simulink model "mrefrobotarm_modified_previous_y_previous_u_previous_ref_pert"  (R2018b)
settings: Solver=FixedStepAuto  StartTime=0.0  StopTime=10  RelTol=1e-3  AbsTol=1e-6
undefined symbols (not defined in the file or in its folder): cc, options
libraries: neural x714, simulink x1
(part 11 of 26)

== system mrefrobotarm_modified_previous_y_previous_u_previous_ref_pert/m=0.01 sd=0.001/Layer 3/Delays 1 ==
  "p{3}" : Inport  PortDimensions=30
      mask Display: e = 0.06;c1 = [120 230 180]/255;c2 = ([120 230 180]+0)/(256+128);c3 = ([120 230 180]+128)/(256+128);patch([0 1 1 0],[0 0 1 1],c1);patch([0 1 1 1-e 1-e 0+e],[0 0 1 1-e 0+e 0+e],c2);patch([0 0 1 1-e 0+e 0+e],[0 1 1 1-e 1-e 0+e],c3);plot([0 1 1 0 0],[0 0 1 1 0]);
  mux : Mux  Inputs=1
      mask Display: e = 0.06;c1 = [120 150 230]/255;c2 = ([120 150 230]+0)/383;c3 = ([120 150 230]+128)/383;patch([0 1 1 0],[0 0 1 1],c1);patch([0 1 1 1-e 1-e 0+e],[0 0 1 1-e 0+e 0+e],c2);patch([0 0 1 1-e 0+e 0+e],[0 1 1 1-e 1-e 0+e],c3);plot([0 1 1 0 0],[0 0 1 1 0]);disp('Mux')
  "pd{3,2}" : Outport
      mask Display: e = 0.06;c1 = [120 230 180]/255;c2 = ([120 230 180]+0)/(256+128);c3 = ([120 230 180]+128)/(256+128);patch([0 1 1 0],[0 0 1 1],c1);patch([0 1 1 1-e 1-e 0+e],[0 0 1 1-e 0+e 0+e],c2);patch([0 0 1 1-e 0+e 0+e],[0 1 1 1-e 1-e 0+e],c3);plot([0 1 1 0 0],[0 0 1 1 0]);
  wires:
  "p{3}"/1 -> mux/1
  mux/1 -> "pd{3,2}"/1

== system mrefrobotarm_modified_previous_y_previous_u_previous_ref_pert/m=0.01 sd=0.001/Layer 3/LW{3,2} ==
  "ad{3,2}" : Inport  PortDimensions=30
      mask Display: e = 0.06;c1 = [120 230 180]/255;c2 = ([120 230 180]+0)/(256+128);c3 = ([120 230 180]+128)/(256+128);patch([0 1 1 0],[0 0 1 1],c1);patch([0 1 1 1-e 1-e 0+e],[0 0 1 1-e 0+e 0+e],c2);patch([0 0 1 1-e 0+e 0+e],[0 1 1 1-e 1-e 0+e],c3);plot([0 1 1 0 0],[0 0 1 1 0]);
  "IW{3,2}(1,:)'" : Constant  Value=[-0.04154814424599621858202880275712232105433940887451171875;-0.0728322351099826847953266906188218854367733001708984375;0.08806929595322621207031943413312546908855438232421875;-0.06181152843373451111208538577557192184031009674072265625;0.05066544886284578275148504644675995223224163055419921875;0.111521575638174275102443289142684079706668853759765625;-0.032112539789640813514548511875545955263078212738037109375;-0.09799349563512209371207717367724399082362651824951171875;0.226222966133449665537824557759449817240238189697265625;-0.0164700269768449925056330584993702359497547149658203125;0.04924878083891880142797248254282749257981777191162109375;-0.31921274972881630294097021760535426437854766845703125;-0.00070955583482500985369190171780928722000680863857269287109375;-0.425499471575058574313032977443072013556957244873046875;-0.30280703571454103961713144599343650043010711669921875;0.020067038188739651227709970271462225355207920074462890625;0.1462301290259256092429751561212469823658466339111328125;0.204274950610219274693690749700181186199188232421875;-0.012345728106829323422743982519023120403289794921875;0.0182316153346177879657208364960752078332006931304931640625;0.1573963175042620010746219350039609707891941070556640625;-0.22786801020675173656826473234104923903942108154296875;-0.06417233312441379677881769794112187810242176055908203125;-0.044370962457045200200145274038732168264687061309814453125;-0.00712369940730364463454815648901785607449710369110107421875;-0.0964821250810107555739847384757013060152530670166015625;0.003950927495288344103163691301006110734306275844573974609375;0.11259508544268000129751072790895705111324787139892578125;-0.1494345742049391356776055772570543922483921051025390625;0.1954892809834287703552035964094102382659912109375]
      mask Display: e = 0.06;c1 = [120 150 230]/255;c2 = ([120 150 230]+0)/383;c3 = ([120 150 230]+128)/383;patch([0 1 1 0],[0 0 1 1],c1);patch([0 1 1 1-e 1-e 0+e],[0 0 1 1-e 0+e 0+e],c2);patch([0 0 1 1-e 0+e 0+e],[0 1 1 1-e 1-e 0+e],c3);plot([0 1 1 0 0],[0 0 1 1 0]);disp('weights');
  Mux : Mux  Inputs=1
      mask Display: e = 0.06;c1 = [120 150 230]/255;c2 = ([120 150 230]+0)/383;c3 = ([120 150 230]+128)/383;patch([0 1 1 0],[0 0 1 1],c1);patch([0 1 1 1-e 1-e 0+e],[0 0 1 1-e 0+e 0+e],c2);patch([0 0 1 1-e 0+e 0+e],[0 1 1 1-e 1-e 0+e],c3);plot([0 1 1 0 0],[0 0 1 1 0]);disp('Mux');
  dotprod1 : neural/Weight Functions/dotprod
  "lz{3,2}" : Outport
      mask Display: e = 0.06;c1 = [120 230 180]/255;c2 = ([120 230 180]+0)/(256+128);c3 = ([120 230 180]+128)/(256+128);patch([0 1 1 0],[0 0 1 1],c1);patch([0 1 1 1-e 1-e 0+e],[0 0 1 1-e 0+e 0+e],c2);patch([0 0 1 1-e 0+e 0+e],[0 1 1 1-e 1-e 0+e],c3);plot([0 1 1 0 0],[0 0 1 1 0]);
  wires:
  "IW{3,2}(1,:)'"/1 -> dotprod1/1
  "ad{3,2}"/1 -> dotprod1/2
  dotprod1/1 -> Mux/1
  Mux/1 -> "lz{3,2}"/1

== system mrefrobotarm_modified_previous_y_previous_u_previous_ref_pert/m=0.1 sd=0.1/Layer 1/Delays 1 ==
  "p{1}" : Inport  PortDimensions=10
      mask Display: e = 0.06;c1 = [120 230 180]/255;c2 = ([120 230 180]+0)/(256+128);c3 = ([120 230 180]+128)/(256+128);patch([0 1 1 0],[0 0 1 1],c1);patch([0 1 1 1-e 1-e 0+e],[0 0 1 1-e 0+e 0+e],c2);patch([0 0 1 1-e 0+e 0+e],[0 1 1 1-e 1-e 0+e],c3);plot([0 1 1 0 0],[0 0 1 1 0]);
  mux : Mux  Inputs=1
      mask Display: e = 0.06;c1 = [120 150 230]/255;c2 = ([120 150 230]+0)/383;c3 = ([120 150 230]+128)/383;patch([0 1 1 0],[0 0 1 1],c1);patch([0 1 1 1-e 1-e 0+e],[0 0 1 1-e 0+e 0+e],c2);patch([0 0 1 1-e 0+e 0+e],[0 1 1 1-e 1-e 0+e],c3);plot([0 1 1 0 0],[0 0 1 1 0]);disp('Mux')
  "pd{1,1}" : Outport
      mask Display: e = 0.06;c1 = [120 230 180]/255;c2 = ([120 230 180]+0)/(256+128);c3 = ([120 230 180]+128)/(256+128);patch([0 1 1 0],[0 0 1 1],c1);patch([0 1 1 1-e 1-e 0+e],[0 0 1 1-e 0+e 0+e],c2);patch([0 0 1 1-e 0+e 0+e],[0 1 1 1-e 1-e 0+e],c3);plot([0 1 1 0 0],[0 0 1 1 0]);
  wires:
  "p{1}"/1 -> mux/1
  mux/1 -> "pd{1,1}"/1

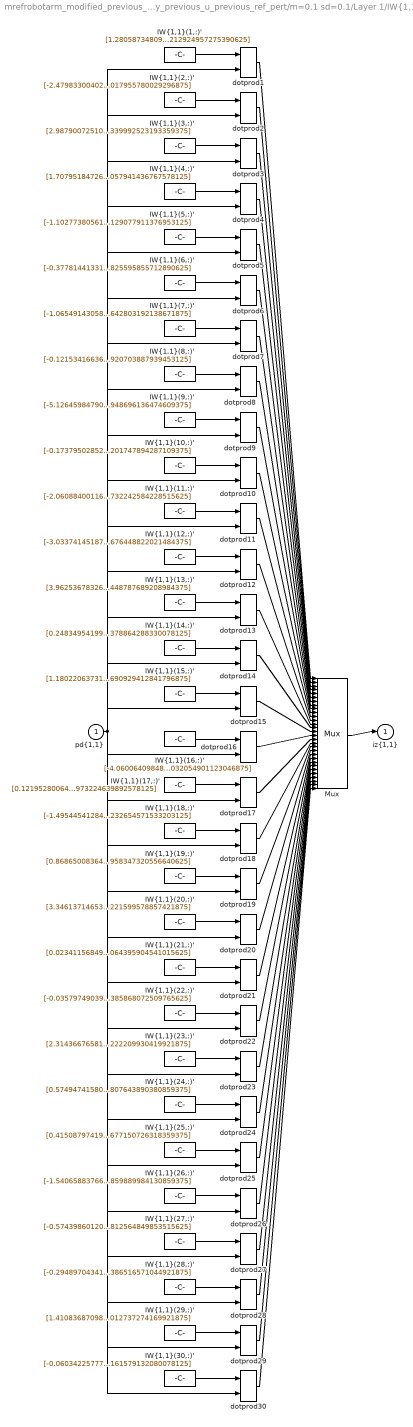
== system mrefrobotarm_modified_previous_y_previous_u_previous_ref_pert/m=0.1 sd=0.1/Layer 1/IW{1,1} ==
  "pd{1,1}" : Inport  PortDimensions=10
      mask Display: e = 0.06;c1 = [120 230 180]/255;c2 = ([120 230 180]+0)/(256+128);c3 = ([120 230 180]+128)/(256+128);patch([0 1 1 0],[0 0 1 1],c1);patch([0 1 1 1-e 1-e 0+e],[0 0 1 1-e 0+e 0+e],c2);patch([0 0 1 1-e 0+e 0+e],[0 1 1 1-e 1-e 0+e],c3);plot([0 1 1 0 0],[0 0 1 1 0]);
  "IW{1,1}(1,:)'" : Constant  Value=[1.2805873480995513258307028081617318093776702880859375;-0.2542545361206982601487425199593417346477508544921875;1.916634122685243912798114251927472651004791259765625;-0.81656061990625838920010437504970468580722808837890625;0.03392905419722232196466649156718631274998188018798828125;-0.56876811356343648373723453914863057434558868408203125;-0.11910574098885444438433722780246171168982982635498046875;-0.10391958490912948931406134533972362987697124481201171875;-0.29880899128876314829739158085430972278118133544921875;0.292440466930168785353316707187332212924957275390625]
      mask Display: e = 0.06;c1 = [120 150 230]/255;c2 = ([120 150 230]+0)/383;c3 = ([120 150 230]+128)/383;patch([0 1 1 0],[0 0 1 1],c1);patch([0 1 1 1-e 1-e 0+e],[0 0 1 1-e 0+e 0+e],c2);patch([0 0 1 1-e 0+e 0+e],[0 1 1 1-e 1-e 0+e],c3);plot([0 1 1 0 0],[0 0 1 1 0]);disp('Weights');
  "IW{1,1}(10,:)'" : Constant  Value=[-0.1737950285201876055030112411259324289858341217041015625;0.39066559991167160159619697878952138125896453857421875;1.4373758788519739315603374052443541586399078369140625;-1.73661635290357008187811516108922660350799560546875;0.95387389217031570698424047805019654333591461181640625;-1.4409587865344988255600355842034332454204559326171875;-1.55823882149022363563517501461319625377655029296875;0.8436188481116324577868681444670073688030242919921875;1.9372499605854283100114798799040727317333221435546875;-0.82246828605585553528811715295887552201747894287109375]
      mask Display: e = 0.06;c1 = [120 150 230]/255;c2 = ([120 150 230]+0)/383;c3 = ([120 150 230]+128)/383;patch([0 1 1 0],[0 0 1 1],c1);patch([0 1 1 1-e 1-e 0+e],[0 0 1 1-e 0+e 0+e],c2);patch([0 0 1 1-e 0+e 0+e],[0 1 1 1-e 1-e 0+e],c3);plot([0 1 1 0 0],[0 0 1 1 0]);disp('Weights');
  "IW{1,1}(11,:)'" : Constant  Value=[-2.06088400116897929592596483416855335235595703125;5.3384112893733348670366467558778822422027587890625;-2.345662279573903052920513800927437841892242431640625;-1.347055891653214931835691459127701818943023681640625;-1.2699131753903916131065443551051430404186248779296875;1.748319175768211497512538699083961546421051025390625;-1.383432805631680917457515533897094428539276123046875;0.96172254081950114823484909720718860626220703125;0.485801400926588911044490259882877580821514129638671875;0.2392142516730272616687358322451473213732242584228515625]
      mask Display: e = 0.06;c1 = [120 150 230]/255;c2 = ([120 150 230]+0)/383;c3 = ([120 150 230]+128)/383;patch([0 1 1 0],[0 0 1 1],c1);patch([0 1 1 1-e 1-e 0+e],[0 0 1 1-e 0+e 0+e],c2);patch([0 0 1 1-e 0+e 0+e],[0 1 1 1-e 1-e 0+e],c3);plot([0 1 1 0 0],[0 0 1 1 0]);disp('Weights');
  "IW{1,1}(12,:)'" : Constant  Value=[-3.033741451879950812298147866385988891124725341796875;1.722438491508440971955451459507457911968231201171875;0.90143553717391478041776053942157886922359466552734375;-1.344538449042689709500564276822842657566070556640625;0.09052755743300877622203870487282983958721160888671875;0.1913628987771903988690525011406862176954746246337890625;0.14300932214249695295649189574760384857654571533203125;0.151940186747806016409612084316904656589031219482421875;0.94345835844083547616634177757077850401401519775390625;-0.489764273889599921485427103107213042676448822021484375]
      mask Display: e = 0.06;c1 = [120 150 230]/255;c2 = ([120 150 230]+0)/383;c3 = ([120 150 230]+128)/383;patch([0 1 1 0],[0 0 1 1],c1);patch([0 1 1 1-e 1-e 0+e],[0 0 1 1-e 0+e 0+e],c2);patch([0 0 1 1-e 0+e 0+e],[0 1 1 1-e 1-e 0+e],c3);plot([0 1 1 0 0],[0 0 1 1 0]);disp('Weights');
  "IW{1,1}(13,:)'" : Constant  Value=[3.962536783267954998422055723494850099086761474609375;-2.296415083745245055979466997087001800537109375;-1.3820553280104583837584186767344363033771514892578125;0.1487002603397468425416860782206640578806400299072265625;0.2557006266995542898001758658210746943950653076171875;0.984039168230778305002104389132000505924224853515625;-1.187417731107363483289418581989593803882598876953125;-0.05262692636122705269752231060920166783034801483154296875;1.51515914985657307312294506118632853031158447265625;1.4552412607900693242157785789459012448787689208984375]
      mask Display: e = 0.06;c1 = [120 150 230]/255;c2 = ([120 150 230]+0)/383;c3 = ([120 150 230]+128)/383;patch([0 1 1 0],[0 0 1 1],c1);patch([0 1 1 1-e 1-e 0+e],[0 0 1 1-e 0+e 0+e],c2);patch([0 0 1 1-e 0+e 0+e],[0 1 1 1-e 1-e 0+e],c3);plot([0 1 1 0 0],[0 0 1 1 0]);disp('Weights');
  "IW{1,1}(14,:)'" : Constant  Value=[0.248349541991651656669404246713384054601192474365234375;-0.57582728691743767512889462523162364959716796875;-0.184076472859580897445397340561612509191036224365234375;0.85012819465897215831517996775801293551921844482421875;-1.8473818086685742656527509097941219806671142578125;2.906900524025082699353106363560073077678680419921875;-1.585858488994206449973489725380204617977142333984375;-1.0106456909323020543212123811827041208744049072265625;2.831929785916387221078593938727863132953643798828125;2.193549040117396931037774265860207378864288330078125]
      mask Display: e = 0.06;c1 = [120 150 230]/255;c2 = ([120 150 230]+0)/383;c3 = ([120 150 230]+128)/383;patch([0 1 1 0],[0 0 1 1],c1);patch([0 1 1 1-e 1-e 0+e],[0 0 1 1-e 0+e 0+e],c2);patch([0 0 1 1-e 0+e 0+e],[0 1 1 1-e 1-e 0+e],c3);plot([0 1 1 0 0],[0 0 1 1 0]);disp('Weights');
  "IW{1,1}(15,:)'" : Constant  Value=[1.180220637311383935497133279568515717983245849609375;-1.68927053848687425130492556490935385227203369140625;-0.205964926311728635521802743824082426726818084716796875;-1.5471983251561602923374039164627902209758758544921875;0.351977698048326625990256388831767253577709197998046875;-0.6072098224125976884124611387960612773895263671875;1.5493999707201970839065552354441024363040924072265625;-0.69103590006371273801732968422584235668182373046875;0.57999299737622589390184657531790435314178466796875;-1.3645924986750219698450337091344408690929412841796875]
      mask Display: e = 0.06;c1 = [120 150 230]/255;c2 = ([120 150 230]+0)/383;c3 = ([120 150 230]+128)/383;patch([0 1 1 0],[0 0 1 1],c1);patch([0 1 1 1-e 1-e 0+e],[0 0 1 1-e 0+e 0+e],c2);patch([0 0 1 1-e 0+e 0+e],[0 1 1 1-e 1-e 0+e],c3);plot([0 1 1 0 0],[0 0 1 1 0]);disp('Weights');
  "IW{1,1}(16,:)'" : Constant  Value=[-4.060064098483632477609717170707881450653076171875;5.38388356599012407599502694210968911647796630859375;3.68619301910720853499014992848969995975494384765625;-4.88748922207302172182608046568930149078369140625;-0.90247651095212899630126912597916088998317718505859375;1.6225975804608470109968720862525515258312225341796875;-1.637634512064228164973656021174974739551544189453125;-0.09186339010871726051821184455548063851892948150634765625;3.27245419173828366865564021281898021697998046875;0.9258097123444766207711609240504913032054901123046875]
      mask Display: e = 0.06;c1 = [120 150 230]/255;c2 = ([120 150 230]+0)/383;c3 = ([120 150 230]+128)/383;patch([0 1 1 0],[0 0 1 1],c1);patch([0 1 1 1-e 1-e 0+e],[0 0 1 1-e 0+e 0+e],c2);patch([0 0 1 1-e 0+e 0+e],[0 1 1 1-e 1-e 0+e],c3);plot([0 1 1 0 0],[0 0 1 1 0]);disp('Weights');
  "IW{1,1}(17,:)'" : Constant  Value=[0.1219528006431145616961231326058623380959033966064453125;0.1872910402036450927543143052389496006071567535400390625;0.509418702105558285353481551283039152622222900390625;-0.60283822874881487496878662568633444607257843017578125;-0.2219694780550395540874575317502603866159915924072265625;0.05471067471573611007418236340527073480188846588134765625;0.56696203361768071626869414103566668927669525146484375;-0.2352711824755020497690338743268512189388275146484375;-0.1887878443087820656831610222070594318211078643798828125;0.45594999319895557210458036934142000973224639892578125]
      mask Display: e = 0.06;c1 = [120 150 230]/255;c2 = ([120 150 230]+0)/383;c3 = ([120 150 230]+128)/383;patch([0 1 1 0],[0 0 1 1],c1);patch([0 1 1 1-e 1-e 0+e],[0 0 1 1-e 0+e 0+e],c2);patch([0 0 1 1-e 0+e 0+e],[0 1 1 1-e 1-e 0+e],c3);plot([0 1 1 0 0],[0 0 1 1 0]);disp('Weights');
  "IW{1,1}(18,:)'" : Constant  Value=[-1.49544541284982646089929403387941420078277587890625;1.439427397485050885705959444749169051647186279296875;0.4193611643381485176718115326366387307643890380859375;-0.15855287177854859859138514366350136697292327880859375;-0.1703669236121354568780361660174094140529632568359375;-0.401336265385540180705703505736892111599445343017578125;0.0160570609236108975681478483465980389155447483062744140625;0.044377601880198402906074761631316505372524261474609375;-0.046548292109242106473487865514471195638179779052734375;-0.04353185958281031997518795151336234994232654571533203125]
      mask Display: e = 0.06;c1 = [120 150 230]/255;c2 = ([120 150 230]+0)/383;c3 = ([120 150 230]+128)/383;patch([0 1 1 0],[0 0 1 1],c1);patch([0 1 1 1-e 1-e 0+e],[0 0 1 1-e 0+e 0+e],c2);patch([0 0 1 1-e 0+e 0+e],[0 1 1 1-e 1-e 0+e],c3);plot([0 1 1 0 0],[0 0 1 1 0]);disp('Weights');
  "IW{1,1}(19,:)'" : Constant  Value=[0.86865008364028983844917775059002451598644256591796875;-1.13188806710383715881107491441071033477783203125;-0.7564355691741797560467830408015288412570953369140625;1.1174434936096317994014270880143158137798309326171875;-0.55981213857717904147648368962109088897705078125;0.51122790846354659866079828134388662874698638916015625;0.128545851201630700888500768996891565620899200439453125;0.2178297237053006540907773569415439851582050323486328125;-0.53417121039822024197718519644695334136486053466796875;-0.14284975311470449188533393680700100958347320556640625]
      mask Display: e = 0.06;c1 = [120 150 230]/255;c2 = ([120 150 230]+0)/383;c3 = ([120 150 230]+128)/383;patch([0 1 1 0],[0 0 1 1],c1);patch([0 1 1 1-e 1-e 0+e],[0 0 1 1-e 0+e 0+e],c2);patch([0 0 1 1-e 0+e 0+e],[0 1 1 1-e 1-e 0+e],c3);plot([0 1 1 0 0],[0 0 1 1 0]);disp('Weights');
  "IW{1,1}(2,:)'" : Constant  Value=[-2.479833004021121833915231036371551454067230224609375;1.350245472571808047490549142821691930294036865234375;-1.9952646111225467162597624337649904191493988037109375;0.93355365506831844424340260957251302897930145263671875;-1.094158035372273740648552120546810328960418701171875;0.0191609773696901457273877866782640921883285045623779296875;0.1756186691672878830150494877671007998287677764892578125;-2.34933052038085321555627160705626010894775390625;-1.10733659534758199782800147659145295619964599609375;1.2836568437066642189847698318772017955780029296875]
      mask Display: e = 0.06;c1 = [120 150 230]/255;c2 = ([120 150 230]+0)/383;c3 = ([120 150 230]+128)/383;patch([0 1 1 0],[0 0 1 1],c1);patch([0 1 1 1-e 1-e 0+e],[0 0 1 1-e 0+e 0+e],c2);patch([0 0 1 1-e 0+e 0+e],[0 1 1 1-e 1-e 0+e],c3);plot([0 1 1 0 0],[0 0 1 1 0]);disp('Weights');
  "IW{1,1}(20,:)'" : Constant  Value=[3.346137146534363449035254234331659972667694091796875;-2.99226479377508969292875917744822800159454345703125;-0.27853125410092849367771350443945266306400299072265625;-0.2936235295146953916400889283977448940277099609375;0.68507743992347058803460413400898687541484832763671875;-2.025831743657712902262346688075922429561614990234375;0.5529546928099247082855072221718728542327880859375;1.409680177963652969452823526808060705661773681640625;0.454782287777185711963312542138737626373767852783203125;-1.5525800409894336961968974719638936221599578857421875]
      mask Display: e = 0.06;c1 = [120 150 230]/255;c2 = ([120 150 230]+0)/383;c3 = ([120 150 230]+128)/383;patch([0 1 1 0],[0 0 1 1],c1);patch([0 1 1 1-e 1-e 0+e],[0 0 1 1-e 0+e 0+e],c2);patch([0 0 1 1-e 0+e 0+e],[0 1 1 1-e 1-e 0+e],c3);plot([0 1 1 0 0],[0 0 1 1 0]);disp('Weights');
  "IW{1,1}(21,:)'" : Constant  Value=[0.0234115684929011268200493844915399677120149135589599609375;0.08943294477851189416828248113233712501823902130126953125;-0.320287324815201113192841830823454074561595916748046875;-0.792896733454647506533774503623135387897491455078125;1.29209875341960156447385088540613651275634765625;0.150087356378403258272413722806959412992000579833984375;-0.262326301140124729105451706345775164663791656494140625;0.61821001174065293159998191185877658426761627197265625;0.143886038068708865811373698306852020323276519775390625;-0.13316750628405371603690809934050776064395904541015625]
      mask Display: e = 0.06;c1 = [120 150 230]/255;c2 = ([120 150 230]+0)/383;c3 = ([120 150 230]+128)/383;patch([0 1 1 0],[0 0 1 1],c1);patch([0 1 1 1-e 1-e 0+e],[0 0 1 1-e 0+e 0+e],c2);patch([0 0 1 1-e 0+e 0+e],[0 1 1 1-e 1-e 0+e],c3);plot([0 1 1 0 0],[0 0 1 1 0]);disp('Weights');
  "IW{1,1}(22,:)'" : Constant  Value=[-0.035797490394503105048951141498037031851708889007568359375;-0.0424545549412682909906635586594347842037677764892578125;0.54593328012475905719469437826774083077907562255859375;-0.1650756208409074332621457870118319988250732421875;-0.2404094021352118637491201980083133094012737274169921875;-0.3064715566776283761640797820291481912136077880859375;0.3468534155097040549975417889072559773921966552734375;0.1192427048713752546493793715853826142847537994384765625;0.22432601366557236577392586696078069508075714111328125;0.10331540330113798964450921857860521413385868072509765625]
      mask Display: e = 0.06;c1 = [120 150 230]/255;c2 = ([120 150 230]+0)/383;c3 = ([120 150 230]+128)/383;patch([0 1 1 0],[0 0 1 1],c1);patch([0 1 1 1-e 1-e 0+e],[0 0 1 1-e 0+e 0+e],c2);patch([0 0 1 1-e 0+e 0+e],[0 1 1 1-e 1-e 0+e],c3);plot([0 1 1 0 0],[0 0 1 1 0]);disp('Weights');
  "IW{1,1}(23,:)'" : Constant  Value=[2.314366765815626170166297015384770929813385009765625;-1.1101450297759998253610547180869616568088531494140625;-0.1532681700664846047299505471528391353785991668701171875;2.241799932360196923042394701042212545871734619140625;-1.76097399523195452530899274279363453388214111328125;-0.76677560057442395446969385375268757343292236328125;-0.0750766427257393009764285807250416837632656097412109375;0.691372661769566132505815403419546782970428466796875;0.553847748207481505033911162172444164752960205078125;0.280210372870193236138902648235671222209930419921875]
      mask Display: e = 0.06;c1 = [120 150 230]/255;c2 = ([120 150 230]+0)/383;c3 = ([120 150 230]+128)/383;patch([0 1 1 0],[0 0 1 1],c1);patch([0 1 1 1-e 1-e 0+e],[0 0 1 1-e 0+e 0+e],c2);patch([0 0 1 1-e 0+e 0+e],[0 1 1 1-e 1-e 0+e],c3);plot([0 1 1 0 0],[0 0 1 1 0]);disp('Weights');
  "IW{1,1}(24,:)'" : Constant  Value=[0.57494741580222419319312621155404485762119293212890625;-1.1856082139566301858479846487171016633510589599609375;-0.271410503358321342215475624470855109393596649169921875;-0.211871891244287346989239040340180508792400360107421875;1.817753405389981313788894112803973257541656494140625;0.0583367822218641418619000660328310914337635040283203125;-0.78196938745817068383558989808079786598682403564453125;0.59968833856100778323394706603721715509891510009765625;0.99671673070357791335283081934903748333454132080078125;-0.319158999411923272049307342967949807643890380859375]
      mask Display: e = 0.06;c1 = [120 150 230]/255;c2 = ([120 150 230]+0)/383;c3 = ([120 150 230]+128)/383;patch([0 1 1 0],[0 0 1 1],c1);patch([0 1 1 1-e 1-e 0+e],[0 0 1 1-e 0+e 0+e],c2);patch([0 0 1 1-e 0+e 0+e],[0 1 1 1-e 1-e 0+e],c3);plot([0 1 1 0 0],[0 0 1 1 0]);disp('Weights');
  "IW{1,1}(25,:)'" : Constant  Value=[0.415087974199574161193737609210074879229068756103515625;-2.032224148951469633317401530803181231021881103515625;-0.729443051610334070034014075645245611667633056640625;1.163530402489732384907483719871379435062408447265625;-1.704018173223377008440593272098340094089508056640625;1.751571810301567833079161573550663888454437255859375;0.01436361471635065611973658405986498109996318817138671875;0.64333357270231827929052315084845758974552154541015625;-1.0562449817232335558259137542336247861385345458984375;-0.4783853710178502804950539939454756677150726318359375]
      mask Display: e = 0.06;c1 = [120 150 230]/255;c2 = ([120 150 230]+0)/383;c3 = ([120 150 230]+128)/383;patch([0 1 1 0],[0 0 1 1],c1);patch([0 1 1 1-e 1-e 0+e],[0 0 1 1-e 0+e 0+e],c2);patch([0 0 1 1-e 0+e 0+e],[0 1 1 1-e 1-e 0+e],c3);plot([0 1 1 0 0],[0 0 1 1 0]);disp('Weights');
  "IW{1,1}(26,:)'" : Constant  Value=[-1.540658837668528402531364918104372918605804443359375;-0.1977184904290689437811323614369030110538005828857421875;1.9098446091703367155645310049294494092464447021484375;-1.4716519993128167609341971910907886922359466552734375;-0.63883709882729744489182621691725216805934906005859375;1.16195036328898737565396004356443881988525390625;-0.319199179979961999986670662110554985702037811279296875;-0.0048271673965746553225386605845415033400058746337890625;1.715497983651685931505426196963526308536529541015625;0.743417601979400100020711761317215859889984130859375]
      mask Display: e = 0.06;c1 = [120 150 230]/255;c2 = ([120 150 230]+0)/383;c3 = ([120 150 230]+128)/383;patch([0 1 1 0],[0 0 1 1],c1);patch([0 1 1 1-e 1-e 0+e],[0 0 1 1-e 0+e 0+e],c2);patch([0 0 1 1-e 0+e 0+e],[0 1 1 1-e 1-e 0+e],c3);plot([0 1 1 0 0],[0 0 1 1 0]);disp('Weights');
  "IW{1,1}(27,:)'" : Constant  Value=[-0.5743986012093824644608730523032136261463165283203125;0.796090033369809102481440277188085019588470458984375;-1.733752597693637209630423967610113322734832763671875;1.7117482137752226822868806266342289745807647705078125;3.060308332219837001986206814763136208057403564453125;1.1745625648314612643474674769095145165920257568359375;-1.3120930290553418640087102176039479672908782958984375;-0.53794869288603652801583621112513355910778045654296875;-0.317071161047647376296509946769219823181629180908203125;-0.9834298498250986231283832239569164812564849853515625]
      mask Display: e = 0.06;c1 = [120 150 230]/255;c2 = ([120 150 230]+0)/383;c3 = ([120 150 230]+128)/383;patch([0 1 1 0],[0 0 1 1],c1);patch([0 1 1 1-e 1-e 0+e],[0 0 1 1-e 0+e 0+e],c2);patch([0 0 1 1-e 0+e 0+e],[0 1 1 1-e 1-e 0+e],c3);plot([0 1 1 0 0],[0 0 1 1 0]);disp('Weights');
  "IW{1,1}(28,:)'" : Constant  Value=[-0.294897043412329917799752365681342780590057373046875;1.8977784660868459720717282834812067449092864990234375;3.246290478544198609966997537412680685520172119140625;-3.246824205937119511844457520055584609508514404296875;-1.49777372582910306419989865389652550220489501953125;-0.10289159011012405375851130884257145226001739501953125;-0.5747446838745104980006317418883554637432098388671875;-5.09856544124092270209303023875690996646881103515625;-3.539096579875632198053381216595880687236785888671875;-1.3660043585555861067604155323351733386516571044921875]
      mask Display: e = 0.06;c1 = [120 150 230]/255;c2 = ([120 150 230]+0)/383;c3 = ([120 150 230]+128)/383;patch([0 1 1 0],[0 0 1 1],c1);patch([0 1 1 1-e 1-e 0+e],[0 0 1 1-e 0+e 0+e],c2);patch([0 0 1 1-e 0+e 0+e],[0 1 1 1-e 1-e 0+e],c3);plot([0 1 1 0 0],[0 0 1 1 0]);disp('Weights');
  "IW{1,1}(29,:)'" : Constant  Value=[1.4108368709849063993289064455893822014331817626953125;-1.61095130575996137167749111540615558624267578125;-2.1911739816554263171610728022642433643341064453125;2.886239792272073056977887972607277333736419677734375;1.0387796064558993958115706846001558005809783935546875;-1.4221551496886923882101427807356230914592742919921875;-0.094203809960493545272441906490712426602840423583984375;-0.48026117694161485349724216575850732624530792236328125;1.1864207388350391791931315310648642480373382568359375;0.08576824055511149402786230666606570594012737274169921875]
      mask Display: e = 0.06;c1 = [120 150 230]/255;c2 = ([120 150 230]+0)/383;c3 = ([120 150 230]+128)/383;patch([0 1 1 0],[0 0 1 1],c1);patch([0 1 1 1-e 1-e 0+e],[0 0 1 1-e 0+e 0+e],c2);patch([0 0 1 1-e 0+e 0+e],[0 1 1 1-e 1-e 0+e],c3);plot([0 1 1 0 0],[0 0 1 1 0]);disp('Weights');
  "IW{1,1}(3,:)'" : Constant  Value=[2.98790072510856763443598538287915289402008056640625;-2.633425635020457900026258357684127986431121826171875;0.170700864782778516381966937842662446200847625732421875;-0.9740642374937940051182749812141992151737213134765625;-0.4226810397158276000340038081048987805843353271484375;0.3079465072150588955679495484218932688236236572265625;0.354941071904679772419655137127847410738468170166015625;0.66817914084442875388702987038413994014263153076171875;-0.299491382907496994647544852341525256633758544921875;1.747008725905569548331186524592339992523193359375]
      mask Display: e = 0.06;c1 = [120 150 230]/255;c2 = ([120 150 230]+0)/383;c3 = ([120 150 230]+128)/383;patch([0 1 1 0],[0 0 1 1],c1);patch([0 1 1 1-e 1-e 0+e],[0 0 1 1-e 0+e 0+e],c2);patch([0 0 1 1-e 0+e 0+e],[0 1 1 1-e 1-e 0+e],c3);plot([0 1 1 0 0],[0 0 1 1 0]);disp('Weights');
  "IW{1,1}(30,:)'" : Constant  Value=[-0.06034225777085043540548525697886361740529537200927734375;0.79781773960256308075855713468627072870731353759765625;1.3071249578309311889512400739477016031742095947265625;-1.55212975494818916644135242677293717861175537109375;0.8377230118391458812965311153675429522991180419921875;-1.889119016922179650208590828697197139263153076171875;0.7410448396540283422240236177458427846431732177734375;1.143342016458946286405762293725274503231048583984375;-3.605371472350964889841407057247124612331390380859375;-1.7740694787859319081491094038938172161579132080078125]
      mask Display: e = 0.06;c1 = [120 150 230]/255;c2 = ([120 150 230]+0)/383;c3 = ([120 150 230]+128)/383;patch([0 1 1 0],[0 0 1 1],c1);patch([0 1 1 1-e 1-e 0+e],[0 0 1 1-e 0+e 0+e],c2);patch([0 0 1 1-e 0+e 0+e],[0 1 1 1-e 1-e 0+e],c3);plot([0 1 1 0 0],[0 0 1 1 0]);disp('Weights');
  "IW{1,1}(4,:)'" : Constant  Value=[1.70795184726016469056730784359388053417205810546875;-3.07831928143786281992788644856773316860198974609375;-1.80334062323873123290240982896648347377777099609375;2.07278852389255607846507700742222368717193603515625;-0.09508658249651313898453963702195324003696441650390625;0.56128334038252780668898367366637103259563446044921875;0.382298565969543091558335845547844655811786651611328125;-0.09223075395815945320965312248517875559628009796142578125;-0.78102192941804571280073332673055119812488555908203125;-0.01264461482980636271300500794723120634444057941436767578125]
      mask Display: e = 0.06;c1 = [120 150 230]/255;c2 = ([120 150 230]+0)/383;c3 = ([120 150 230]+128)/383;patch([0 1 1 0],[0 0 1 1],c1);patch([0 1 1 1-e 1-e 0+e],[0 0 1 1-e 0+e 0+e],c2);patch([0 0 1 1-e 0+e 0+e],[0 1 1 1-e 1-e 0+e],c3);plot([0 1 1 0 0],[0 0 1 1 0]);disp('Weights');
  "IW{1,1}(5,:)'" : Constant  Value=[-1.102773805616038327315209244261495769023895263671875;2.423613884872370061174251532065682113170623779296875;-1.4714769357123456128277894094935618340969085693359375;2.6826906922715494374642730690538883209228515625;0.199112432453587284708618199147167615592479705810546875;-1.8564017530623229124131512435269542038440704345703125;-0.413724421313545753786655723160947673022747039794921875;0.67504674409264120438223244491382502019405364990234375;0.05156579303588627871679506142754689790308475494384765625;-0.2189514774450145584427929179582861252129077911376953125]
      mask Display: e = 0.06;c1 = [120 150 230]/255;c2 = ([120 150 230]+0)/383;c3 = ([120 150 230]+128)/383;patch([0 1 1 0],[0 0 1 1],c1);patch([0 1 1 1-e 1-e 0+e],[0 0 1 1-e 0+e 0+e],c2);patch([0 0 1 1-e 0+e 0+e],[0 1 1 1-e 1-e 0+e],c3);plot([0 1 1 0 0],[0 0 1 1 0]);disp('Weights');
  "IW{1,1}(6,:)'" : Constant  Value=[-0.377814413310031016468570896904566325247287750244140625;0.437245561324330400676529961856431327760219573974609375;-0.37200441352368629477354033951996825635433197021484375;0.2882898323214033720063298460445366799831390380859375;0.1614505662292759768927652430647867731750011444091796875;-0.12882361717835999481707176528288982808589935302734375;-0.088022315595546796185288940250757150352001190185546875;-0.435647010295977910043774272708105854690074920654296875;0.53537279854982211535485703279846347868442535400390625;0.10426477846615213318504089556881808675825595855712890625]
      mask Display: e = 0.06;c1 = [120 150 230]/255;c2 = ([120 150 230]+0)/383;c3 = ([120 150 230]+128)/383;patch([0 1 1 0],[0 0 1 1],c1);patch([0 1 1 1-e 1-e 0+e],[0 0 1 1-e 0+e 0+e],c2);patch([0 0 1 1-e 0+e 0+e],[0 1 1 1-e 1-e 0+e],c3);plot([0 1 1 0 0],[0 0 1 1 0]);disp('Weights');
  "IW{1,1}(7,:)'" : Constant  Value=[-1.0654914305821423514686330236145295202732086181640625;1.9281642007601786925619080648175440728664398193359375;-2.4681473271198246521862529334612190723419189453125;1.52384317988985973357785042026080191135406494140625;0.42706121614108105699614270633901469409465789794921875;0.436990354971589223254113676375709474086761474609375;0.246994258256146625996052534901537001132965087890625;1.3144601358611527341935243384796194732189178466796875;-1.254608881296326305943011902854777872562408447265625;-0.70568441913970303414060936120222322642803192138671875]
      mask Display: e = 0.06;c1 = [120 150 230]/255;c2 = ([120 150 230]+0)/383;c3 = ([120 150 230]+128)/383;patch([0 1 1 0],[0 0 1 1],c1);patch([0 1 1 1-e 1-e 0+e],[0 0 1 1-e 0+e 0+e],c2);patch([0 0 1 1-e 0+e 0+e],[0 1 1 1-e 1-e 0+e],c3);plot([0 1 1 0 0],[0 0 1 1 0]);disp('Weights');
  "IW{1,1}(8,:)'" : Constant  Value=[-0.121534166367048890311508557715569622814655303955078125;0.82007157853148981985214049927890300750732421875;-1.6831216261787391719195738915004767477512359619140625;0.97013957263959393895191851697745732963085174560546875;0.25773636895133378299505011455039493739604949951171875;0.26618267249609151026135123174753971397876739501953125;-0.42911401641808399887167979613877832889556884765625;-0.42012714648697435659840948574128560721874237060546875;0.4338105500457880570053248447948135435581207275390625;0.4925519079354974127937794037279672920703887939453125]
      mask Display: e = 0.06;c1 = [120 150 230]/255;c2 = ([120 150 230]+0)/383;c3 = ([120 150 230]+128)/383;patch([0 1 1 0],[0 0 1 1],c1);patch([0 1 1 1-e 1-e 0+e],[0 0 1 1-e 0+e 0+e],c2);patch([0 0 1 1-e 0+e 0+e],[0 1 1 1-e 1-e 0+e],c3);plot([0 1 1 0 0],[0 0 1 1 0]);disp('Weights');
  "IW{1,1}(9,:)'" : Constant  Value=[-5.1264598479079506176958602736704051494598388671875;2.65819019981378179551256835111416876316070556640625;5.085771341342894658055229228921234607696533203125;-4.191239159301868966167603502981364727020263671875;-0.56802519257872841063061741806450299918651580810546875;0.8211703615580689952224702210514806210994720458984375;1.2509404859962101053127980776480399072170257568359375;-0.1606546807912663521467067084813606925308704376220703125;-2.255001000090772311779119263519532978534698486328125;-1.2084777631717855683746165595948696136474609375]
      mask Display: e = 0.06;c1 = [120 150 230]/255;c2 = ([120 150 230]+0)/383;c3 = ([120 150 230]+128)/383;patch([0 1 1 0],[0 0 1 1],c1);patch([0 1 1 1-e 1-e 0+e],[0 0 1 1-e 0+e 0+e],c2);patch([0 0 1 1-e 0+e 0+e],[0 1 1 1-e 1-e 0+e],c3);plot([0 1 1 0 0],[0 0 1 1 0]);disp('Weights');
  Mux : Mux  Inputs=30
      mask Display: e = 0.06;c1 = [120 150 230]/255;c2 = ([120 150 230]+0)/383;c3 = ([120 150 230]+128)/383;patch([0 1 1 0],[0 0 1 1],c1);patch([0 1 1 1-e 1-e 0+e],[0 0 1 1-e 0+e 0+e],c2);patch([0 0 1 1-e 0+e 0+e],[0 1 1 1-e 1-e 0+e],c3);plot([0 1 1 0 0],[0 0 1 1 0]);disp('Mux');
  dotprod{1..30} (30 alike) : neural/Weight Functions/dotprod
  "iz{1,1}" : Outport
      mask Display: e = 0.06;c1 = [120 230 180]/255;c2 = ([120 230 180]+0)/(256+128);c3 = ([120 230 180]+128)/(256+128);patch([0 1 1 0],[0 0 1 1],c1);patch([0 1 1 1-e 1-e 0+e],[0 0 1 1-e 0+e 0+e],c2);patch([0 0 1 1-e 0+e 0+e],[0 1 1 1-e 1-e 0+e],c3);plot([0 1 1 0 0],[0 0 1 1 0]);
  wires:
  "IW{1,1}(1,:)'"/1 -> dotprod1/1
  "pd{1,1}"/1 -> dotprod1/2, dotprod2/2, dotprod3/2, dotprod4/2, dotprod5/2, dotprod6/2, dotprod7/2, dotprod8/2, dotprod9/2, dotprod10/2, dotprod11/2, dotprod12/2, dotprod13/2, dotprod14/2, dotprod15/2, dotprod16/2, dotprod17/2, dotprod18/2, dotprod19/2, dotprod20/2, dotprod21/2, dotprod22/2, dotprod23/2, dotprod24/2, dotprod25/2, dotprod26/2, dotprod27/2, dotprod28/2, dotprod29/2, dotprod30/2
  dotprod1/1 -> Mux/1
  "IW{1,1}(2,:)'"/1 -> dotprod2/1
  dotprod2/1 -> Mux/2
  "IW{1,1}(3,:)'"/1 -> dotprod3/1
  dotprod3/1 -> Mux/3
  "IW{1,1}(4,:)'"/1 -> dotprod4/1
  dotprod4/1 -> Mux/4
  "IW{1,1}(5,:)'"/1 -> dotprod5/1
  dotprod5/1 -> Mux/5
  "IW{1,1}(6,:)'"/1 -> dotprod6/1
  dotprod6/1 -> Mux/6
  "IW{1,1}(7,:)'"/1 -> dotprod7/1
  dotprod7/1 -> Mux/7
  "IW{1,1}(8,:)'"/1 -> dotprod8/1
  dotprod8/1 -> Mux/8
  "IW{1,1}(9,:)'"/1 -> dotprod9/1
  dotprod9/1 -> Mux/9
  "IW{1,1}(10,:)'"/1 -> dotprod10/1
  dotprod10/1 -> Mux/10
  "IW{1,1}(11,:)'"/1 -> dotprod11/1
  dotprod11/1 -> Mux/11
  "IW{1,1}(12,:)'"/1 -> dotprod12/1
  dotprod12/1 -> Mux/12
  "IW{1,1}(13,:)'"/1 -> dotprod13/1
  dotprod13/1 -> Mux/13
  "IW{1,1}(14,:)'"/1 -> dotprod14/1
  dotprod14/1 -> Mux/14
  "IW{1,1}(15,:)'"/1 -> dotprod15/1
  dotprod15/1 -> Mux/15
  "IW{1,1}(16,:)'"/1 -> dotprod16/1
  dotprod16/1 -> Mux/16
  "IW{1,1}(17,:)'"/1 -> dotprod17/1
  dotprod17/1 -> Mux/17
  "IW{1,1}(18,:)'"/1 -> dotprod18/1
  dotprod18/1 -> Mux/18
  "IW{1,1}(19,:)'"/1 -> dotprod19/1
  dotprod19/1 -> Mux/19
  "IW{1,1}(20,:)'"/1 -> dotprod20/1
  dotprod20/1 -> Mux/20
  "IW{1,1}(21,:)'"/1 -> dotprod21/1
  dotprod21/1 -> Mux/21
  "IW{1,1}(22,:)'"/1 -> dotprod22/1
  dotprod22/1 -> Mux/22
  "IW{1,1}(23,:)'"/1 -> dotprod23/1
  dotprod23/1 -> Mux/23
  "IW{1,1}(24,:)'"/1 -> dotprod24/1
  dotprod24/1 -> Mux/24
  "IW{1,1}(25,:)'"/1 -> dotprod25/1
  dotprod25/1 -> Mux/25
  "IW{1,1}(26,:)'"/1 -> dotprod26/1
  dotprod26/1 -> Mux/26
  "IW{1,1}(27,:)'"/1 -> dotprod27/1
  dotprod27/1 -> Mux/27
  "IW{1,1}(28,:)'"/1 -> dotprod28/1
  dotprod28/1 -> Mux/28
  "IW{1,1}(29,:)'"/1 -> dotprod29/1
  dotprod29/1 -> Mux/29
  "IW{1,1}(30,:)'"/1 -> dotprod30/1
  dotprod30/1 -> Mux/30
  Mux/1 -> "iz{1,1}"/1

== system mrefrobotarm_modified_previous_y_previous_u_previous_ref_pert/m=0.1 sd=0.1/Layer 2/Delays 1 ==
  "p{2}" : Inport  PortDimensions=30
      mask Display: e = 0.06;c1 = [120 230 180]/255;c2 = ([120 230 180]+0)/(256+128);c3 = ([120 230 180]+128)/(256+128);patch([0 1 1 0],[0 0 1 1],c1);patch([0 1 1 1-e 1-e 0+e],[0 0 1 1-e 0+e 0+e],c2);patch([0 0 1 1-e 0+e 0+e],[0 1 1 1-e 1-e 0+e],c3);plot([0 1 1 0 0],[0 0 1 1 0]);
  mux : Mux  Inputs=1
      mask Display: e = 0.06;c1 = [120 150 230]/255;c2 = ([120 150 230]+0)/383;c3 = ([120 150 230]+128)/383;patch([0 1 1 0],[0 0 1 1],c1);patch([0 1 1 1-e 1-e 0+e],[0 0 1 1-e 0+e 0+e],c2);patch([0 0 1 1-e 0+e 0+e],[0 1 1 1-e 1-e 0+e],c3);plot([0 1 1 0 0],[0 0 1 1 0]);disp('Mux')
  "pd{2,1}" : Outport
      mask Display: e = 0.06;c1 = [120 230 180]/255;c2 = ([120 230 180]+0)/(256+128);c3 = ([120 230 180]+128)/(256+128);patch([0 1 1 0],[0 0 1 1],c1);patch([0 1 1 1-e 1-e 0+e],[0 0 1 1-e 0+e 0+e],c2);patch([0 0 1 1-e 0+e 0+e],[0 1 1 1-e 1-e 0+e],c3);plot([0 1 1 0 0],[0 0 1 1 0]);
  wires:
  "p{2}"/1 -> mux/1
  mux/1 -> "pd{2,1}"/1
